simulink model "sedemo_aggregation"  (Simulink 7.5)
settings: Solver=VariableStepDiscrete  StartTime=0.0  StopTime=20.0  MaxStep=inf  RelTol=1e-3
undefined symbols (not defined in the file or in its folder): des_attributefunction_support, des_figposition
libraries: simeventsattributes2 x6, simeventsserver1 x6, simeventssink1 x3, simeventsgenerators1 x3, simulink x3, simeventsentitymanage1 x1, simeventsinfo x1, simeventstranslate1 x1
settings Model: Creator=The MathWorks Inc.  ExtModeAutoUpdateStatusClock=off
settings DataIOCC: SaveOutput=off  SignalLogging=off  SaveTime=off
settings OptimizationCC: InitFltsAndDblsToZero=on
settings DebuggingCC: AlgebraicLoopMsg=error  SolverPrmCheckMsg=none  StrictBusMsg=Warning
settings SimEventsCC: propDiagAttribOutput=1  propDiagFcnCallOutput=1  propDiagStatOutput=0

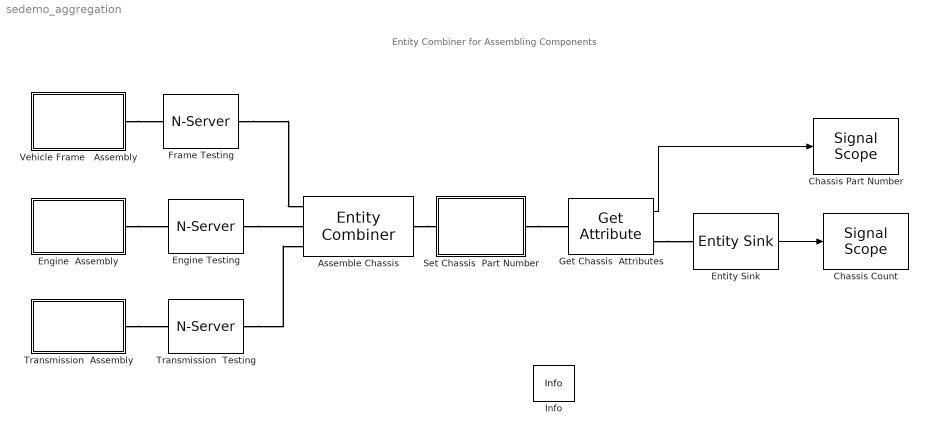
== system sedemo_aggregation ==
  note: Entity Combiner for Assembling Components
  Assemble Chassis : simeventsentitymanage1/Entity Combiner  Priority=1  SystemSampleTime=-1  NumberInputPorts=3  RetainComponentEntities=on  AttributeAccessibility=on  TimerAccessibility=on  AttributeCopied=on  TimerCopied=on  StatNumberDeparted=Off  EvaluatedNumPorts=3
  "Chassis Count " : simeventssink1/Signal Scope  Priority=1  SystemSampleTime=-1  PlotType=Stair  InputType=Signal  NumInputs=1  AttributeNameY=Count  XInputOptionSignal=Event time  XInputOptionEntity=Event time  AttributeNameX=Count  EnableEntityOutport=on  XMin=0  XMax=20  XLimitExceededOption=Stretch axis limits  YLimitExceededOption=Stretch axis limits  AxisGrid=on  AxisLegend=off  LineDisables=""  LineColors=b  LineStyles=-  LineMarkers=.  OpenScopeAtSimStart=on  Title=Chassis Count  YLabel=Count  XLabel=Time  FigurePosition=des_figposition([15,5,22,22])  AxisZoom=off  DataStoreOption=Limited  DataPointsLimit=10000  StatNumberArrived=Off  ShowCountPlotted=off  ShowToolbar=off
      settings: YMin=0  YMax=20
  Chassis Part Number : simeventssink1/Signal Scope  Priority=1  SystemSampleTime=-1  PlotType=Stair  InputType=Signal  NumInputs=1  AttributeNameY=Count  XInputOptionSignal=Event time  XInputOptionEntity=Event time  AttributeNameX=Count  EnableEntityOutport=on  XMin=-0.198  XMax=19.998  XLimitExceededOption=Stretch axis limits  YLimitExceededOption=Stretch axis limits  AxisGrid=on  AxisLegend=off  LineDisables=""  LineColors=b  LineStyles=-  LineMarkers=.  OpenScopeAtSimStart=on  Title=Chassis Part Number  YLabel=Part Number  XLabel=Time  FigurePosition=des_figposition([45,5,22,22])  AxisZoom=off  DataStoreOption=Limited  DataPointsLimit=10000  StatNumberArrived=Off  ShowCountPlotted=off  ShowToolbar=off
      settings: YMin=-0.07  YMax=7.07
  Engine  Assembly : Subsystem
  Engine Testing : simeventsserver1/N-Server  Priority=1  SystemSampleTime=-1  NumberOfServers=1  ServiceTimeFrom=Dialog  ServiceTime=.3  AttributeName=ServiceTime  PriorityServiceCompletion=500  EnableTOPort=off  StatNumberDeparted=Off  StatNumberInBlock=Off  StatPendingEntity=Off  StatNumberPending=Off  StatAverageWait=Off  StatUtilization=Off  StatNumberTimedout=Off
  Entity Sink : simeventssink1/Entity Sink  Priority=1  SystemSampleTime=-1  AvailableForArrivals=on  StatNumberArrived=On
  Frame Testing : simeventsserver1/N-Server  Priority=1  SystemSampleTime=-1  NumberOfServers=1  ServiceTimeFrom=Dialog  ServiceTime=.5  AttributeName=ServiceTime  PriorityServiceCompletion=500  EnableTOPort=off  StatNumberDeparted=Off  StatNumberInBlock=Off  StatPendingEntity=Off  StatNumberPending=Off  StatAverageWait=Off  StatUtilization=Off  StatNumberTimedout=Off
  Get Chassis  Attributes : simeventsattributes2/Get Attribute  Priority=1  DialogController=des_ddg_create  DialogControllerArgs=DataTag12  SystemSampleTime=-1  AttributeName=ChassisPartNumber  AttributeMissing=Error  AttributeDefaultValue=1  AttributeSendTiming=After entity departure  AttributeTreatAsVector=1  StatNumberDeparted=Off  EvaluatedDefaultAttributeValue={[]}
  Info : simeventsinfo/Info  SystemSampleTime=-1
  Set Chassis  Part Number : Subsystem  LoadFcn=des_attributefunction_support(gcb,'LoadFcn');  StartFcn=des_attributefunction_support(gcb,'StartFcn');  mask(Attribute Function){OutputNamePrefix=out_}
      mask prompts: OutputNamePrefix "Prefix name"
      settings: CopyFcn=des_attributefunction_support(gcb,'CopyFcn');  OpenFcn=des_attributefunction_support(gcb,'OpenFcn');  ErrorFcn=des_error_redirect
      mask Display: image(des_iconLoad('attribFunction.jpg'),'center');
  Transmission  Assembly : Subsystem
  Transmission  Testing : simeventsserver1/N-Server  Priority=1  SystemSampleTime=-1  NumberOfServers=1  ServiceTimeFrom=Dialog  ServiceTime=.6  AttributeName=ServiceTime  PriorityServiceCompletion=500  EnableTOPort=off  StatNumberDeparted=Off  StatNumberInBlock=Off  StatPendingEntity=Off  StatNumberPending=Off  StatAverageWait=Off  StatUtilization=Off  StatNumberTimedout=Off
  Vehicle Frame   Assembly : Subsystem
  wires:
  Entity Sink/1 -> "Chassis Count "/1
  Get Chassis  Attributes/1 -> Chassis Part Number/1
  connections:
  Transmission  Assembly/RConn1 -- Transmission  Testing/LConn1
  Engine  Assembly/RConn1 -- Engine Testing/LConn1
  Vehicle Frame   Assembly/RConn1 -- Frame Testing/LConn1
  Frame Testing/RConn1 -- Assemble Chassis/LConn1
  Engine Testing/RConn1 -- Assemble Chassis/LConn2
  Transmission  Testing/RConn1 -- Assemble Chassis/LConn3
  Assemble Chassis/RConn1 -- Set Chassis  Part Number/LConn1
  Set Chassis  Part Number/RConn1 -- Get Chassis  Attributes/LConn1
  Get Chassis  Attributes/RConn1 -- Entity Sink/LConn1

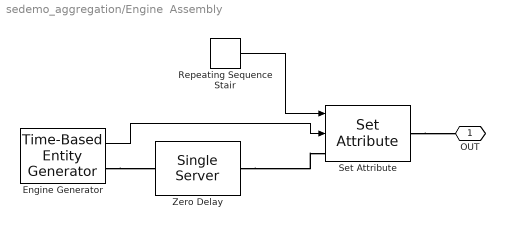
== system sedemo_aggregation/Engine  Assembly ==
  Engine Generator : simeventsgenerators1/Entity Generators/Time-Based Entity Generator  Priority=1  DialogController=des_ddg_create  DialogControllerArgs=DataTag4  SystemSampleTime=-1  GenerateEntitiesUpon=Intergeneration time from dialog  Distribution=Constant  Minimum=0  Maximum=1  Mean=1  InitialSeed=12345  Period=.2  PriorityEntityGeneration=300  GenerateEntityAtSimulationStart=on  ResponseWhenBlocked=Pause generation  ResponseWhenUnblocked=Immediate restart  EntityType=Blank  StatNumberDeparted=On  StatPendingEntity=Off  StatAverageIntergenerationTime=Off
  Repeating Sequence Stair : simulink/Sources/Repeating Sequence Stair  SystemSampleTime=-1  OutValues=[3 4].'  tsamp=3  OutputDataTypeScalingMode=Specify via dialog  OutDataType=float('double')  ConRadixGroup=Best Precision: Vector-wise  OutScaling=2^-12
  Set Attribute : simeventsattributes2/Set Attribute  Priority=1  DialogController=des_ddg_create  DialogControllerArgs=DataTag6  SystemSampleTime=-1  AttributeFrom=Signal port|Signal port  AttributeName=EnginePartNumber|EngineSN  AttributeTreatAsVector=1|1  AttributeValue=1|1  AttributeCreate=on  StatNumberDeparted=Off  EvaluatedAttributeValue={[];[]}
  Zero Delay : simeventsserver1/Single Server  Priority=1  SystemSampleTime=-1  ServiceTimeFrom=Dialog  ServiceTime=0  AttributeName=ServiceTime  PriorityServiceCompletion=1  PermitPreemption=off  SortingAttributeName=PriorityAttributeName  SortingDirection=Ascending  WriteToAttribute=off  ResidualAttributeName=ResidualServiceTime  CreateAttribute=on  EnableTOPort=off  StatNumberDeparted=Off  StatNumberInBlock=Off  StatNumberPreempted=Off  StatPendingEntity=Off  StatAverageWait=Off  StatUtilization=Off  StatNumberTimedout=Off
  OUT : PMIOPort  Port=1  Side=Right
  wires:
  Engine Generator/1 -> Set Attribute/2
  Repeating Sequence Stair/1 -> Set Attribute/1
  connections:
  Engine Generator/RConn1 -- Zero Delay/LConn1
  Set Attribute/RConn1 -- OUT/RConn1
  Zero Delay/RConn1 -- Set Attribute/LConn1

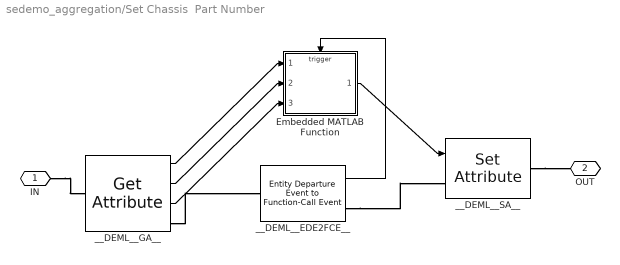
== system sedemo_aggregation/Set Chassis  Part Number ==
  Embedded MATLAB Function : Stateflow chart  TreatAsAtomicUnit=on
      settings: PropExecContextOutsideSubsystem=on
  __DEML__EDE2FCE__ : simeventstranslate1/Entity Departure Event to Function-Call Event  Priority=1  SystemSampleTime=-1  TimingFunctionCallF1=Before entity departure  EnableE1Port=off  EnableF2Port=off  TimingFunctionCallF2=Before entity departure  EnableE2Port=off  StatNumberDeparted=Off  StatNumberF1Calls=Off  StatNumberF2Calls=Off  IsInsideAFB=on
  __DEML__GA__ : simeventsattributes2/Get Attribute  Priority=1  DialogController=des_ddg_create  DialogControllerArgs=DataTag15  SystemSampleTime=-1  AttributeName=FramePartNumber|EnginePartNumber|TransmissionPartNumber  AttributeMissing=Error|Error|Error  AttributeDefaultValue=1|1|1  AttributeSendTiming=Before entity departure|Before entity departure|Before entity departure  AttributeTreatAsVector=1|1|1  StatNumberDeparted=Off  EvaluatedDefaultAttributeValue={[];[];[]}
  __DEML__SA__ : simeventsattributes2/Set Attribute  Priority=1  DialogController=des_ddg_create  DialogControllerArgs=DataTag17  SystemSampleTime=-1  AttributeFrom=Signal port  AttributeName=ChassisPartNumber  AttributeTreatAsVector=1  AttributeValue=1  AttributeCreate=on  StatNumberDeparted=Off  EvaluatedAttributeValue={[]}
  IN : PMIOPort  Port=1  Side=Left
  OUT : PMIOPort  Port=2  Side=Right
  wires:
  __DEML__EDE2FCE__/1 -> Embedded MATLAB Function/Trigger
  __DEML__GA__/1 -> Embedded MATLAB Function/1(FramePartNumber)
  __DEML__GA__/2 -> Embedded MATLAB Function/2(EnginePartNumber)
  __DEML__GA__/3 -> Embedded MATLAB Function/3(TransmissionPartNumber)
  Embedded MATLAB Function/1(out_ChassisPartNumber) -> __DEML__SA__/1
  connections:
  __DEML__SA__/RConn1 -- OUT/RConn1
  IN/RConn1 -- __DEML__GA__/LConn1
  __DEML__GA__/RConn1 -- __DEML__EDE2FCE__/LConn1
  __DEML__EDE2FCE__/RConn1 -- __DEML__SA__/LConn1

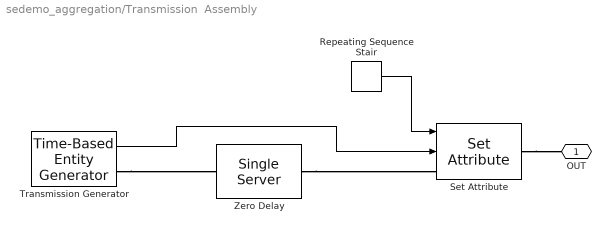
== system sedemo_aggregation/Transmission  Assembly ==
  Repeating Sequence Stair : simulink/Sources/Repeating Sequence Stair  SystemSampleTime=-1  OutValues=[5 5 5 5 6 6 6 6].'  tsamp=3  OutputDataTypeScalingMode=Specify via dialog  OutDataType=float('double')  ConRadixGroup=Best Precision: Vector-wise  OutScaling=2^-12
  Set Attribute : simeventsattributes2/Set Attribute  Priority=1  DialogController=des_ddg_create  DialogControllerArgs=DataTag19  SystemSampleTime=-1  AttributeFrom=Signal port|Signal port  AttributeName=TransmissionPartNumber|TransmissionSN  AttributeTreatAsVector=1|1  AttributeValue=1|1  AttributeCreate=on  StatNumberDeparted=Off  EvaluatedAttributeValue={[];[]}
  Transmission Generator : simeventsgenerators1/Entity Generators/Time-Based Entity Generator  Priority=1  DialogController=des_ddg_create  DialogControllerArgs=DataTag21  SystemSampleTime=-1  GenerateEntitiesUpon=Intergeneration time from dialog  Distribution=Constant  Minimum=0  Maximum=1  Mean=1  InitialSeed=12345  Period=.3  PriorityEntityGeneration=300  GenerateEntityAtSimulationStart=on  ResponseWhenBlocked=Pause generation  ResponseWhenUnblocked=Immediate restart  EntityType=Blank  StatNumberDeparted=On  StatPendingEntity=Off  StatAverageIntergenerationTime=Off
  Zero Delay : simeventsserver1/Single Server  Priority=1  SystemSampleTime=-1  ServiceTimeFrom=Dialog  ServiceTime=0  AttributeName=ServiceTime  PriorityServiceCompletion=1  PermitPreemption=off  SortingAttributeName=PriorityAttributeName  SortingDirection=Ascending  WriteToAttribute=off  ResidualAttributeName=ResidualServiceTime  CreateAttribute=on  EnableTOPort=off  StatNumberDeparted=Off  StatNumberInBlock=Off  StatNumberPreempted=Off  StatPendingEntity=Off  StatAverageWait=Off  StatUtilization=Off  StatNumberTimedout=Off
  OUT : PMIOPort  Port=1  Side=Right
  wires:
  Transmission Generator/1 -> Set Attribute/2
  Repeating Sequence Stair/1 -> Set Attribute/1
  connections:
  Set Attribute/RConn1 -- OUT/RConn1
  Zero Delay/RConn1 -- Set Attribute/LConn1
  Transmission Generator/RConn1 -- Zero Delay/LConn1

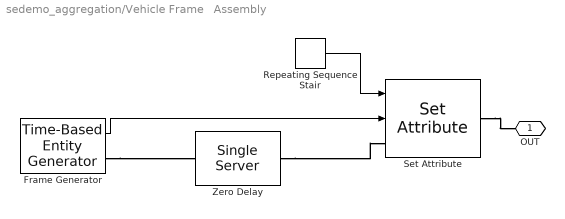
== system sedemo_aggregation/Vehicle Frame   Assembly ==
  Frame Generator : simeventsgenerators1/Entity Generators/Time-Based Entity Generator  Priority=1  DialogController=des_ddg_create  DialogControllerArgs=DataTag25  SystemSampleTime=-1  GenerateEntitiesUpon=Intergeneration time from dialog  Distribution=Constant  Minimum=0  Maximum=1  Mean=1  InitialSeed=12345  Period=.1  PriorityEntityGeneration=300  GenerateEntityAtSimulationStart=on  ResponseWhenBlocked=Pause generation  ResponseWhenUnblocked=Immediate restart  EntityType=Blank  StatNumberDeparted=On  StatPendingEntity=Off  StatAverageIntergenerationTime=Off
  Repeating Sequence Stair : simulink/Sources/Repeating Sequence Stair  SystemSampleTime=-1  OutValues=[1 1 2 2 ].'  tsamp=3  OutputDataTypeScalingMode=Specify via dialog  OutDataType=float('double')  ConRadixGroup=Best Precision: Vector-wise  OutScaling=2^-12
  Set Attribute : simeventsattributes2/Set Attribute  Priority=1  DialogController=des_ddg_create  DialogControllerArgs=DataTag27  SystemSampleTime=-1  AttributeFrom=Signal port|Signal port  AttributeName=FramePartNumber|FrameSN  AttributeTreatAsVector=1|1  AttributeValue=1|1  AttributeCreate=on  StatNumberDeparted=Off  EvaluatedAttributeValue={[];[]}
  Zero Delay : simeventsserver1/Single Server  Priority=1  SystemSampleTime=-1  ServiceTimeFrom=Dialog  ServiceTime=0  AttributeName=ServiceTime  PriorityServiceCompletion=1  PermitPreemption=off  SortingAttributeName=PriorityAttributeName  SortingDirection=Ascending  WriteToAttribute=off  ResidualAttributeName=ResidualServiceTime  CreateAttribute=on  EnableTOPort=off  StatNumberDeparted=Off  StatNumberInBlock=Off  StatNumberPreempted=Off  StatPendingEntity=Off  StatAverageWait=Off  StatUtilization=Off  StatNumberTimedout=Off
  OUT : PMIOPort  Port=1  Side=Right
  wires:
  Frame Generator/1 -> Set Attribute/2
  Repeating Sequence Stair/1 -> Set Attribute/1
  connections:
  Set Attribute/RConn1 -- OUT/RConn1
  Zero Delay/RConn1 -- Set Attribute/LConn1
  Frame Generator/RConn1 -- Zero Delay/LConn1

== matlab function Set Chassis Part Number/Embedded MATLAB Function ==
  data: FramePartNumber input double; out_ChassisPartNumber output double; EnginePartNumber input double; TransmissionPartNumber input double
  events: trigger input FUNCTION_CALL_EVENT
function out_ChassisPartNumber  = fcn(FramePartNumber,EnginePartNumber,...
                                        TransmissionPartNumber)
                                        
%This function derives a chassis part number from the part numbers of the 
%constituent frame, engine and transmission parts. This value is assigned 
%to the newly created ChassisPartNumber attribute.
%

bias = 1;
out_ChassisPartNumber = ((FramePartNumber-1)*1) + ... 
                    ((EnginePartNumber -3)*2) + ...
                    ((TransmissionPartNumber - 5) * 4) + bias;
